simulink model "oncalisma301_2"  (R2020a)
settings: Solver=VariableStepAuto  StartTime=0.0  StopTime=10.0  RelTol=1e-3
settings Model: Creator=nartc  LastModifiedBy=nartc

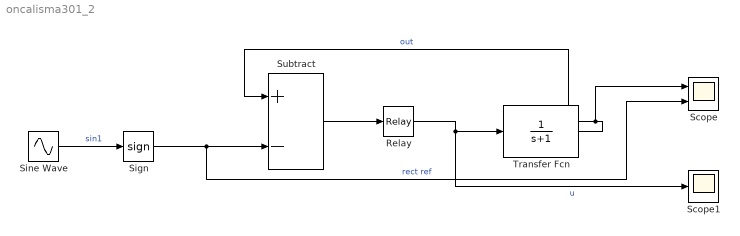
== system oncalisma301_2 ==
  Relay : Relay  OnSwitchValue=1  OffSwitchValue=-1  OnOutputValue=-12  OffOutputValue=12
  Scope : Scope  NumInputPorts=2
  Scope1 : Scope
  Sign : Signum
  Sine Wave : Sin  Frequency=2*pi*0.1  SampleTime=0
  Subtract : Sum  Inputs=+-
  Transfer Fcn : TransferFcn  Denominator=[1 1]
  wires:
  Relay/1 -> Scope1/1, Transfer Fcn/1  "u"
  Subtract/1 -> Relay/1
  Transfer Fcn/1 -> Subtract/1, Scope/1  "out"
  Sine Wave/1 -> Sign/1  "sin1"
  Sign/1 -> Scope/2, Subtract/2  "rect ref"
